simulink model "powertrain_control_3"  (R2026a)
settings: Solver=VariableStepAuto  StopTime=100  AbsTol=1e-3
PostLoadFcn:
  | num_fric_surf = 6;
  | eff_tor_rad = 0.4;
  | engagement_area = 0.0025;
  | peak_normal = 0.55;
  | fric_coeff = 0.5;
  | clutchRise = 0.1;
  | velTol = 1e-3;
  | pressThresh = 0.05;
  | p0 = 20e5;
undefined symbols (not defined in the file): sigbuilder_block
libraries: sdl_lib x13, fl_lib x11, nesl_utility x10
Description:
  | Copyright 2017-2026 The MathWorks, Inc.
settings Model: Creator=smiller  LastModifiedBy=smiller
settings ConfigComp: CovMetricSettings=dswe
settings SimscapeCC: SimscapeNormalizeSystem=off  SimscapeNominalValues="[{\"value\":\"1\",\"unit\":\"A\"},{\"value\":\"1\",\"unit\":\"bar\"},{\"value\":\"1\",\"unit\":\"cm^2\"},{\"value\":\"1\",\"unit\":\"cm^3/s\"},{\"value\":\"1\",\"unit\":\"kJ/kg\"},{\"value\":\"1\",\"unit\":\"kW\"},{\"value\":\"1\",\"unit\":\"l\"},{\"value\":\"1\",\"unit\":\"N\"},{\"value\":\"1\",\"unit\":\"N*m\"},{\"value\":\"1\",\"unit\":\"V\"}]"

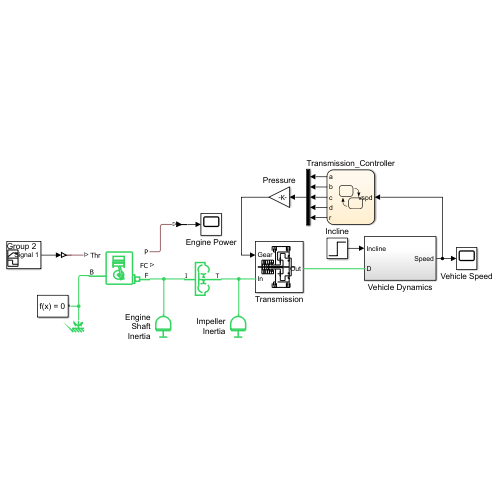
[thumbnail: Simulink's stored preview of the top-level diagram]
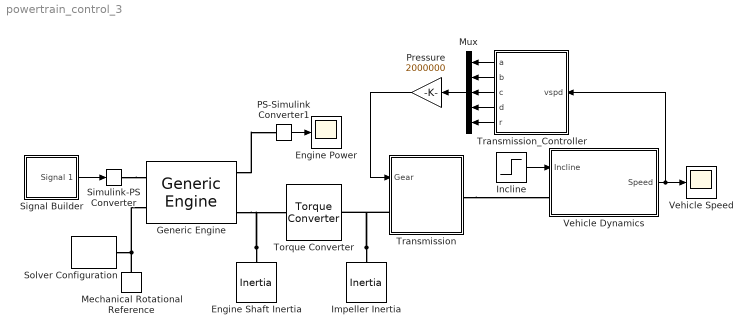
== system powertrain_control_3 ==
  Engine Shaft Inertia : fl_lib/Mechanical/Rotational Elements/Inertia  inertia=0.2 kg*m^2  num_ports=foundation.enum.numPorts2.one  w_specify=on  w_priority=High  w=800 rpm  w_nominal_specify=off  w_nominal_value=1  w_nominal_unit=rad/s  t_specify=off  t_priority=High  t=0 N*m  t_nominal_specify=off  t_nominal_value=1  t_nominal_unit=N*m
  Engine Power : Scope
      settings: ActiveDisplayYMinimum=-18750.18434  ActiveDisplayYMaximum=168751.65909
  Generic Engine : sdl_lib/Engines & Motors/Generic Engine  input_type=sdl.enum.GenericEngineInputType.NormalizedThrottle  model_parameterization=1  engine_type=1  Trq_max=380 N*m  w_Trq_max=4300 rpm  P_max=1.5e+5 W  w_P_max=4.5e+3 rpm  w_max=6e+3 rpm  w_min=500 rpm  w_tab=[ 500 1000 2e+3 3e+3 4e+3 5e+3 6e+3 7e+3 ] rpm  trq_tab=[ 380 380 380 380 350 280 200 80 ] N*m  pwr_tab=[ 2e+4 4e+4 7.8e+4 1.2e+5 1.45e+5 1.48e+5 1.25e+5 6e+4 ] W  interp_method=1  w_thr=100 rpm  model_inertia=0  inertia=1 kg*m^2  initial_velocity=800 rpm  model_time_constant=0  time_constant=0.2 s  initial_normalized_throttle=0  fc_model=1  fc_per_rev=25 mg/rev  fc_w_tab=[ 1000 2e+3 3e+3 4e+3 5e+3 6e+3 ] rpm  fc_trq_tab=[ 0 80 160 200 240 320 360 400 ] N*m  fc_tab=[ 0.5 0.9 1.4 1.6 1.9 2.7 3.4 4.4; 1 1.7 2.7 3.1 3.6 5 6 7.4; 1.4 2.7 4 4.8 5.6 7.5 8.5 10.5; 2 3.6 5.8 6.7 8 10.4 11.7 13.3; 2.5 4.8 7.9 9.4 10.8 14 16.2 18.6; 3.1 6 10.3 11.9 13.8 18.4 22 26.5 ] g/s  bmep_tab=[ 0 250 500 625 750 1000 1.15e+3 1.25e+3 ] kPa  bsfc_tab=[ 410 380 300 280 270 290 320 380; 410 370 290 270 260 270 285 320; 415 380 290 275 265 270 270 300; 420 390 310 290 285 280 280 285; 430 410 340 320 310 300 310 320; 450 430 370 340 330 330 350 380 ] g/hr/kW  fc_interp_method=1  displaced_volume=400 cm^3  rev_per_cycle=2  idle_speed=0  idle_speed_reference=1000 rpm  tau_controller=1 s  idle_w_thr=1 rpm  redline=0  redline_speed=5000 rpm  tau_redline=1 s  redline_w_thr=1 rpm
  Impeller Inertia : fl_lib/Mechanical/Rotational Elements/Inertia  inertia=1 kg*m^2  num_ports=foundation.enum.numPorts2.one  w_specify=on  w_priority=High  w=0 rpm  w_nominal_specify=off  w_nominal_value=1  w_nominal_unit=rad/s  t_specify=off  t_priority=High  t=0 N*m  t_nominal_specify=off  t_nominal_value=1  t_nominal_unit=N*m
  Incline : Step  Time=5  FinalValue=20  SampleTime=0
  Mechanical Rotational Reference : fl_lib/Mechanical/Rotational Elements/Mechanical Rotational Reference
  Mux : Mux  Inputs=5
  PS-Simulink Converter1 : nesl_utility/PS-Simulink Converter  PhysicalDomain=network_engine_domain  SubClassName=ps_output  LeftPortType=input  RightPortType=output  PseudoPeriodic=off  Frequencies=[]  VectorFormat=1-D array  Unit=W  AffineConversion=off
  Pressure : Gain  Gain=2000000
  Signal Builder : Subsystem  Tag=STV Subsys  LoadFcn=sigbuilder_block('load');  StartFcn=sigbuilder_block('start');  StopFcn=sigbuilder_block('stop');  ClipboardFcn=sigbuilder_block('clipboard');  mask(Sigbuilder block){tuvar=[0:10]}
      mask help: Simulink:masks:SigbuilderBlock_MD
      mask init:
      | if ~strcmp(get_param(bdroot(gcbh),'SimulationStatus'),'stopped') tuvar = sigbuilder_block('maskInit'); end
      settings: CopyFcn=sigbuilder_block('copy');  DeleteFcn=sigbuilder_block('delete');  ModelCloseFcn=sigbuilder_block('modelClose');  PreSaveFcn=sigbuilder_block('preSave');  PauseFcn=sigbuilder_block('pause');  ContinueFcn=sigbuilder_block('continue');  NameChangeFcn=sigbuilder_block('namechange');  OpenFcn=sigbuilder_block('open',[53.4 199.8 550.8 400.2 ]);  CloseFcn=sigbuilder_block('close');
      mask Display: plot(0, 0, 100, 100,[2, 2, 32, 32, 2], [68, 8, 8, 68, 68],[32, 2], [38, 38], [32, 19, 2],[53, 60, 44], [32, 17, 17, 2],[16, 16, 31, 31]);txt = getActiveGroup(gcbh);text(2, 100, txt,'verticalAlignment', 'top');
  Simulink-PS Converter : nesl_utility/Simulink-PS Converter  PhysicalDomain=network_engine_domain  SubClassName=ps_input  LeftPortType=input  RightPortType=output  PseudoPeriodic=off  Frequencies=[]  NoiseDistribution=none  NoiseParameters=[]  Unit=1  AffineConversion=off  FilteringAndDerivatives=zero  SimscapeFilterOrder=1  InputFilterTimeConstant=0.001  UdotUserProvided=1
  Solver Configuration : nesl_utility/Solver Configuration  PhysicalDomain=network_engine_domain  SubClassName=solver  LeftPortType=input  RightPortType=generic  Tones=[]  Harmonics=[]  SimulateNoise=off  Profile=off  UseLocalSampling=off  EnableSwitchedLinearOptims=on  FrequencyDomain=off  UseCCode=off  RelTol=0.001  AbsTol=1e-06  MinStep=1e-09  ToWorkspace=off  RevertToSquareIcSolve=off  NumHomotopyIterations=100  PhasorMode=off  PhasorModeNumHarmonics=1  ConsistencySolver=NEWTON_FTOL  CanonicalOrdering=UNORDERED  OptimizeIntermediates=UNOPTIMIZED  IndexReductionMethod=DerivativeReplacement  DoDC=off  ResidualTolerance=1e-9  ConsistencyTolSource=GLOBAL  ConsistencyAbsTol=0.001  ConsistencyRelTol=0.001  ConsistencyTolFactor=0.001  UseLocalSolver=off  LocalSolverChoice=NE_BACKWARD_EULER_ADVANCER  ResolveIndetEquations=on  FunctionEvalNumThread=1  LocalSolverSampleTime=.001  DoFixedCost=off  MaxNonlinIter=3  MaxModeIter=2  ComputeImpulses=off  ImpulseIterations=2  LinearAlgebra=Sparse  LinearAlgebraNumThread=0  EquationFormulation=NE_TIME_EF  DelaysMemoryBudget=1024  AutomaticFiltering=on  FilteringTimeConstant=0.001  PartitionStorageMethod=AS_NEEDED  PartitionMemoryBudget=1024  PartitionMethod=FAST  MultibodyUseLocalSolver=off  MultibodyLocalSolverChoice=ODE1  MultibodyLocalSolverSampleTime=0.001
  Torque Converter : sdl_lib/Couplings & Drives/Torque Converter  coast_mode_modeling=sdl.enum.torqueConverterContinuousTwomode.continuous  SR_drive_tlu=[0, .5, .6, .7, .8, .87, .92, .94, .96, .97, 1]  TR_drive_tlu=[2.232, 1.5462, 1.4058, 1.2746, 1.1528, 1.0732, 1.0192, 1, 1, 1, 1]  CF_drive_tlu=1e-4 * [.72558, .66322, .63463, .59042, .51331, .4144, .29287, .22444, .12186, .04386, 0] m*N/rpm^2  SR_coast_tlu=[0, .5, .6, .7, .8, .87, .92, .94, .96, .97, 1]  CF_coast_tlu=1e-4 * [.5079, .4643, .4442, .4133, .3593, .2901, .205, .1571, .0853, .0307, 0] m*N/rpm^2  iniMode=sdl.enum.torqueConverterInitialMode.drive  delta_w=1 rpm  n_vector=[ 0 0.5 0.6 0.7 0.8 0.81 0.82 0.83 0.84 0.85 0.86 0.87 0.88 0.89 0.9 0.92 0.94 0.96 0.97 ]  trq_vector=[ 2.232 1.5462 1.4058 1.2746 1.1528 1.1412 1.1296 1.1181 1.1067 1.0955 1.0843 1.0732 1.0622 1.0513 1.0405 1.0192 0.9983 0.9983 0.9983 ]  cf_vector_parameterization=1  cf_vector_reference_speed=1  cf_vector=[ 12.2938 12.8588 13.1452 13.6285 14.6163 14.7747 14.9516 15.1502 15.3748 15.6309 15.9253 16.2675 16.6698 17.1492 17.7298 19.3503 22.1046 29.9986 50 ] (rad/s)/(N*m)^0.5  cf_vector_sq=[ 0.006615999999999999 0.006048 0.005787 0.005384 0.004681 0.004581 0.004473 0.004357 0.00423 0.004093 0.003943 0.003779 0.003599 0.0034 0.003181 0.002671 0.002047 0.001111 4e-4 ] N*m/(rad/s)^2  interp_method=simscape.enum.interpolation.linear  extrap_method=simscape.enum.extrapolation.linear  model_lag=0  tau=0.02 s  initial_trq_ratio=0
  Transmission : Subsystem  Tag=PublishSubsystem  mask(CR-CR 4-Speed){}
      mask help: This is a template for a CR-CR 4-speed transmission. Copy it to your model, open it as a subsystem, and modify it for your use.
      settings: OpenFcn=open_system(gcbh,'force');
      mask Help: web(drive_help);
      mask Display:
      | % Icon data
      | Icon.x1 = [-1.3 -1.1 -1.1 -1 -1 -1 -0.9 -0.9 -0.9 -0.8 -0.8];
      | Icon.x1_1 = [-0.8 -0.7 -0.7 -0.7 -0.6 -0.6 -0.6 -0.5 -0.5 -0.5];
      | Icon.y1 = [0 0 0.15 0.15 0.05 0.15 0.15 0.05 0.15 0.15 0.05];
      | Icon.y1_1 =[0.15 0.15 0.05 0.15 0.15 0.07 0.15 0.15 0.07 0.15];
      | Icon.x2 = [-1.05 -1.05 -0.95 -0.95 -0.95 0.3];
      | Icon.y2 = [0.08   0     0     0.08  0    0];
      | Icon.x3 = [-0.85 -0.85 -0.75 -0.75 -0.75 0 0 -0.3 -0.3  0.3];
      | Icon.y3 = [0.08 0.02 0.02 0.08 0.02 0.02 0.15 0.15 0.33 0.33];
      | Icon.x3_1 = [-0.65 -0.65 -0.55 -0.55 -0.55 -0.4];
      | Icon.y3_1 = [0.1    0.05  0.05  0.1   0.05 0.05];
      | Icon.x4 = [-0.2 -0.1 -0.15 -0.15 -0.2 -0.1];
      | Icon.y4 = [0.12 0.12 0.12 0.18 0.18 0.18];
      | Icon.x5 = [-0.2 -0.1 -0.1 -0.15 -0.15 -0.4 -0.4];
      | Icon.y5 = [0.1 0.1 0.1 0.1 0.05 0.05 0.4];
      | Icon.x6 = [-0.2 -0.1 -0.15 -0.15 0.1 0.1 0.4 0.4];
      | Icon.y6 = [0.20 0.20 0.20 0.3 0.3 0.19 0.19 0];
      | Icon.x7 = [0.3 0.3 0.25 0.35];
      | Icon.y7 = [0 0.13 0.13 0.13];
      | Icon.x8 = [0.25 0.35 0.3 0.3 0.25 0.35];
      | Icon.y8 = [0.15 0.15 0.15 0.23 0.23 0.23];
      | Icon.x9 = [0.25 0.35 0.3 0.3];
      | Icon.y9 = [0.25 0.25 0.25 0.40];
      | Icon.x10 = [0.25 0.25 0.35 0.35 0.35 0.15 0.15 0.15];
      | Icon.y10 = [0.35 0.45 0.45 0.35 0.45 0.45 0.35 0.45];
      | Icon.x11 = [0.2 0.2];
      | Icon.y11 = [0.33 0.40];
      | Icon.x12 = [0.4 0.6];
      | Icon.y12 = [0 0];
      | Icon.x13 = [-0.45 -0.45 -0.35 -0.35 -0.35 -0.55 -0.55];
      | Icon.y13 = [0.35 0.45 0.45 0.35 0.45 0.45 0.35];
      | Icon.x14 = [-0.4 -0.5 -0.5];
      | Icon.y14 = [0.33 0.33 0.4];
      | Icon.x15 = [-0.5 0.35];
      | Icon.y15 = [0.45 0.45];
      | Icon.x16 = [-1.3 -1.1 -1.1 -1 -1 -1 -0.9 -0.9 ];
      | Icon.x16_1 = [-0.9 -0.8 -0.8 -0.8 -0.7 -0.7 -0.7 -0.6];
      | Icon.x16_2 = [-0.6 -0.6 -0.5 -0.5 -0.5];
      | Icon.y16 = [0 0 -0.15 -0.15 -0.05 -0.15 -0.15 -0.05];
      | Icon.y16_1 = [-0.15 -0.15 -0.05 -0.15 -0.15 -0.05 -0.15 -0.15];
      | Icon.y16_2 = [-0.07 -0.15 -0.15 -0.07 -0.15];
      | Icon.x17 = [-1.05 -1.05 -0.95 -0.95 -0.95 0.3];
      | Icon.y17 = [-0.08 0 0 -0.08 0 0];
      | Icon.x18 = [-0.85 -0.85 -0.75 -0.75 -0.75 0 0 -0.3];
      | Icon.x18_1 = [-0.3  0.3];
      | Icon.x18_2 = [-0.65 -0.65 -0.55 -0.55 -0.55 -0.4];
      | Icon.y18 = [-0.08 -0.02 -0.02 -0.08 -0.02 -0.02 -0.15 -0.15];
      | Icon.y18_1 = [-0.33 -0.33];
      | Icon.y18_2 = [-0.1 -0.05 -0.05 -0.1 -0.05 -0.05];
      | Icon.x19 = [-0.2 -0.1 -0.15 -0.15 -0.2 -0.1];
      | Icon.y19 = [-0.12 -0.12 -0.12 -0.18 -0.18 -0.18];
      | Icon.x20 = [-0.2 -0.1 -0.1 -0.15 -0.15 -0.4 -0.4];
      | Icon.y20 = [-0.1 -0.1 -0.1 -0.1 -0.05 -0.05 -0.4];
      | Icon.x21 = [-0.2 -0.1 -0.15 -0.15 0.1 0.1 0.4 0.4];
      | Icon.y21 = [-0.20 -0.20 -0.20 -0.3 -0.3 -0.19 -0.19 0];
      | Icon.x22 = [0.3 0.3 0.25 0.35];
      | Icon.y22 = [0 -0.13 -0.13 -0.13];
      | Icon.x23 = [0.25 0.35 0.3 0.3 0.25 0.35];
      | Icon.y23 = [-0.15 -0.15 -0.15 -0.23 -0.23 -0.23];
      | Icon.x24 = [0.25 0.35 0.3 0.3];
      | Icon.y24 = [-0.25 -0.25 -0.25 -0.40];
      | Icon.x25 = [0.25 0.25 0.35 0.35 0.35 0.15 0.15 0.15];
      | Icon.y25 = [-0.35 -0.45 -0.45 -0.35 -0.45 -0.45 -0.35 -0.45];
      | Icon.x26 = [0.2 0.2];
      | Icon.y26 = [-0.33 -0.40];
      | Icon.x27 = [-0.45 -0.45 -0.35 -0.35 -0.35 -0.55 -0.55];
      | Icon.y27 = [-0.35 -0.45 -0.45 -0.35 -0.45 -0.45 -0.35];
      | Icon.x28 = [-0.4 -0.5 -0.5];
      | Icon.y28 = [-0.33 -0.33 -0.4];
      | Icon.x29 = [-0.5 0.35];
      | Icon.y29 = [-0.45 -0.45];
      | % Bounding box
      | Icon.LowerLeftx = -1.4;
      | Icon.LowerLefty = -0.55;
      | Icon.UpperRightx = 1.0;
      | Icon.UpperRighty = 0.55;
      | 
      | plot(Icon.x1,Icon.y1);
      | plot(Icon.x1_1,Icon.y1_1);
      | plot(Icon.x2,Icon.y2);
      | plot(Icon.x3,Icon.y3);
      | plot(Icon.x3_1,Icon.y3_1);
      | plot(Icon.x4,Icon.y4);
      | plot(Icon.x5,Icon.y5);
      | plot(Icon.x6,Icon.y6);
      | plot(Icon.x7,Icon.y7);
      | plot(Icon.x8,Icon.y8);
      | plot(Icon.x9,Icon.y9);
      | plot(Icon.x10,Icon.y10);
      | plot(Icon.x11,Icon.y11);
      | plot(Icon.x12,Icon.y12);
      | plot(Icon.x13,Icon.y13);
      | plot(Icon.x14,Icon.y14);
      | plot(Icon.x15,Icon.y15);
      | plot(Icon.x16,Icon.y16);
      | plot(Icon.x16_1,Icon.y16_1);
      | plot(Icon.x16_2,Icon.y16_2);
      | plot(Icon.x17,Icon.y17);
      | plot(Icon.x18,Icon.y18);
      | plot(Icon.x18_1,Icon.y18_1);
      | plot(Icon.x18_2,Icon.y18_2);
      | plot(Icon.x19,Icon.y19);
      | plot(Icon.x20,Icon.y20);
      | plot(Icon.x21,Icon.y21);
      | plot(Icon.x22,Icon.y22);
      | plot(Icon.x23,Icon.y23);
      | plot(Icon.x24,Icon.y24);
      | plot(Icon.x25,Icon.y25);
      | plot(Icon.x26,Icon.y26);
      | plot(Icon.x27,Icon.y27);
      | plot(Icon.x28,Icon.y28);
      | plot(Icon.x29,Icon.y29);
      | 
      | plot(Icon.LowerLeftx,Icon.LowerLefty);
      | plot(Icon.UpperRightx,Icon.UpperRighty);
  Transmission_Controller : Stateflow chart  TreatAsAtomicUnit=on
  Vehicle Dynamics : Subsystem
  Vehicle Speed : Scope
      settings: ActiveDisplayYMinimum=-12.57055  ActiveDisplayYMaximum=113.13493
  wires:
  Vehicle Dynamics/1(Speed) -> Transmission_Controller/1(vspd), Vehicle Speed/1
  PS-Simulink Converter1/1 -> Engine Power/1
  Incline/1 -> Vehicle Dynamics/1(Incline)
  Transmission_Controller/1(a) -> Mux/1
  Transmission_Controller/2(b) -> Mux/2
  Transmission_Controller/3(c) -> Mux/3
  Transmission_Controller/4(d) -> Mux/4
  Transmission_Controller/5(r) -> Mux/5
  Mux/1 -> Pressure/1
  Pressure/1 -> Transmission/1(Gear)
  Signal Builder/1(Signal 1) -> Simulink-PS Converter/1
  connections:
  Solver Configuration/RConn1 -- Mechanical Rotational Reference/LConn1 -- Generic Engine/LConn2
  Impeller Inertia/LConn1 -- Transmission/LConn1 -- Torque Converter/RConn1
  Engine Shaft Inertia/LConn1 -- Torque Converter/LConn1 -- Generic Engine/RConn3
  Transmission/RConn1 -- Vehicle Dynamics/LConn1
  Generic Engine/RConn1 -- PS-Simulink Converter1/LConn1
  Simulink-PS Converter/RConn1 -- Generic Engine/LConn1

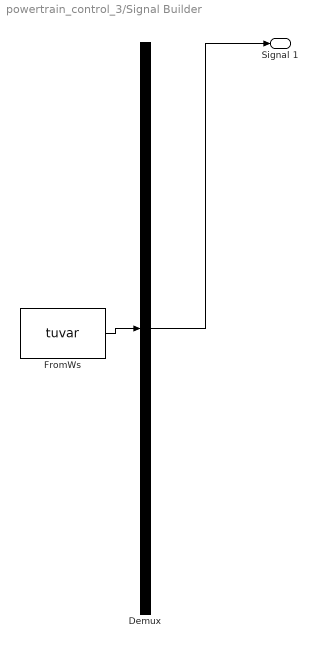
== system powertrain_control_3/Signal Builder ==
  Demux : Demux  Tag=STV Demux  Outputs=1
      settings: DisplayOption=none
  FromWs : FromWorkspace  Tag=STV FromWs  VariableName=tuvar
      SigBuilderData=|
      | common.afterFinalStr = 'Extrapolate'
      | common.sampleTime = 0
      | dataSet(1).timeRange = [0 100]
      | dataSet(1).name = 'Group 1'
      | dataSet(2).timeRange = [0 100]
      | dataSet(2).name = 'Group 2'
      | sbobj.Groups(1).Name = 'Group 1'
      | sbobj.Groups(1).Signals.Name = 'Signal 1'
      | sbobj.Groups(1).Signals.XData = [0 100]
      | sbobj.Groups(1).Signals.YData = [1 1]
      | sbobj.Groups(1).TimeRange = [0 100]
      | sbobj.Groups(2).Name = 'Group 2'
      | sbobj.Groups(2).Signals.Name = 'Signal 1'
      | sbobj.Groups(2).Signals.XData = [0 40 40 100]
      | sbobj.Groups(2).Signals.YData = [0.5 0.5 1 1]
      | sbobj.Groups(2).TimeRange = [0 100]
  Signal 1 : Outport  Tag=STV Outport  VectorParamsAs1DForOutWhenUnconnected=off
  wires:
  Demux/1 -> Signal 1/1
  FromWs/1 -> Demux/1

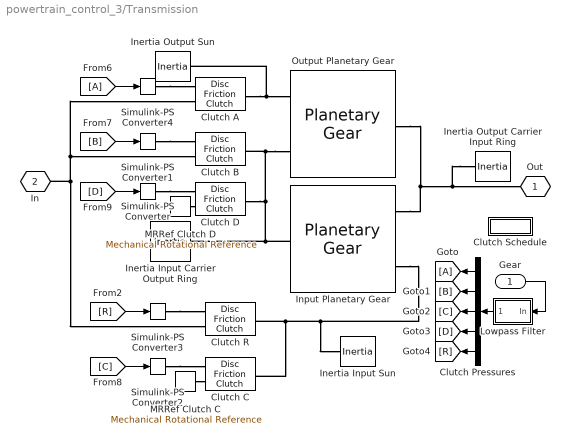
== system powertrain_control_3/Transmission ==
  Gear : Inport
  Clutch Pressures : Demux  Outputs=5
  Clutch A : sdl_lib/Clutches/Disc Friction Clutch  geometry_model=1  r_eff=eff_tor_rad m  d_o=0.15 m  d_i=0.1 m  nS=num_fric_surf  piston_area=engagement_area m^2  unidirectional=0  friction_model=1  mu_w_vector=[ 0 0.1 0.2 0.3 0.4 0.5 1 2 5 10 100 1000 ] rad/s  temperature_TLU=[280.0, 300.0, 320.0] K  mu_static=peak_normal  mu_static_vector=[0.4, 0.38, 0.36]  mu_coulomb=fric_coeff  mu_coulomb_vector=[ 0.29 0.28 0.26 0.22 0.21 0.2 0.2 0.19 0.19 0.19 0.19 0.19 ]  mu_coulomb_temp_vector=[0.3, 0.28, 0.25]  mu_coulomb_matrix=[0.34, 0.32, 0.3; 0.3, 0.28, 0.25; 0.25, 0.2, 0.15]  mu_interp_method=1  mu_extrap_method=1  d_f=1  w_tol=velTol rad/s  pressure_min=pressThresh*p0 Pa  mu_visc=0 N*m/(rad/s)  initial_state_locked=1  thermal_mass=25 kJ/K  T_init=300 K
  Clutch B : sdl_lib/Clutches/Disc Friction Clutch  geometry_model=1  r_eff=eff_tor_rad m  d_o=0.15 m  d_i=0.1 m  nS=num_fric_surf  piston_area=engagement_area m^2  unidirectional=0  friction_model=1  mu_w_vector=[ 0 0.1 0.2 0.3 0.4 0.5 1 2 5 10 100 1000 ] rad/s  temperature_TLU=[280.0, 300.0, 320.0] K  mu_static=peak_normal  mu_static_vector=[0.4, 0.38, 0.36]  mu_coulomb=fric_coeff  mu_coulomb_vector=[ 0.29 0.28 0.26 0.22 0.21 0.2 0.2 0.19 0.19 0.19 0.19 0.19 ]  mu_coulomb_temp_vector=[0.3, 0.28, 0.25]  mu_coulomb_matrix=[0.34, 0.32, 0.3; 0.3, 0.28, 0.25; 0.25, 0.2, 0.15]  mu_interp_method=1  mu_extrap_method=1  d_f=1  w_tol=velTol rad/s  pressure_min=pressThresh*p0 Pa  mu_visc=0 N*m/(rad/s)  initial_state_locked=0  thermal_mass=25 kJ/K  T_init=300 K
  Clutch C : sdl_lib/Clutches/Disc Friction Clutch  geometry_model=1  r_eff=eff_tor_rad m  d_o=0.15 m  d_i=0.1 m  nS=num_fric_surf  piston_area=engagement_area m^2  unidirectional=0  friction_model=1  mu_w_vector=[ 0 0.1 0.2 0.3 0.4 0.5 1 2 5 10 100 1000 ] rad/s  temperature_TLU=[280.0, 300.0, 320.0] K  mu_static=peak_normal  mu_static_vector=[0.4, 0.38, 0.36]  mu_coulomb=fric_coeff  mu_coulomb_vector=[ 0.29 0.28 0.26 0.22 0.21 0.2 0.2 0.19 0.19 0.19 0.19 0.19 ]  mu_coulomb_temp_vector=[0.3, 0.28, 0.25]  mu_coulomb_matrix=[0.34, 0.32, 0.3; 0.3, 0.28, 0.25; 0.25, 0.2, 0.15]  mu_interp_method=1  mu_extrap_method=1  d_f=1  w_tol=velTol rad/s  pressure_min=pressThresh*p0 Pa  mu_visc=0 N*m/(rad/s)  initial_state_locked=0  thermal_mass=25 kJ/K  T_init=300 K
  Clutch D : sdl_lib/Clutches/Disc Friction Clutch  geometry_model=1  r_eff=eff_tor_rad m  d_o=0.15 m  d_i=0.1 m  nS=num_fric_surf  piston_area=engagement_area m^2  unidirectional=0  friction_model=1  mu_w_vector=[ 0 0.1 0.2 0.3 0.4 0.5 1 2 5 10 100 1000 ] rad/s  temperature_TLU=[280.0, 300.0, 320.0] K  mu_static=peak_normal  mu_static_vector=[0.4, 0.38, 0.36]  mu_coulomb=fric_coeff  mu_coulomb_vector=[ 0.29 0.28 0.26 0.22 0.21 0.2 0.2 0.19 0.19 0.19 0.19 0.19 ]  mu_coulomb_temp_vector=[0.3, 0.28, 0.25]  mu_coulomb_matrix=[0.34, 0.32, 0.3; 0.3, 0.28, 0.25; 0.25, 0.2, 0.15]  mu_interp_method=1  mu_extrap_method=1  d_f=1  w_tol=velTol rad/s  pressure_min=pressThresh*p0 Pa  mu_visc=0 N*m/(rad/s)  initial_state_locked=1  thermal_mass=25 kJ/K  T_init=300 K
  Clutch R : sdl_lib/Clutches/Disc Friction Clutch  geometry_model=1  r_eff=eff_tor_rad m  d_o=0.15 m  d_i=0.1 m  nS=num_fric_surf  piston_area=engagement_area m^2  unidirectional=0  friction_model=1  mu_w_vector=[ 0 0.1 0.2 0.3 0.4 0.5 1 2 5 10 100 1000 ] rad/s  temperature_TLU=[280.0, 300.0, 320.0] K  mu_static=peak_normal  mu_static_vector=[0.4, 0.38, 0.36]  mu_coulomb=fric_coeff  mu_coulomb_vector=[ 0.29 0.28 0.26 0.22 0.21 0.2 0.2 0.19 0.19 0.19 0.19 0.19 ]  mu_coulomb_temp_vector=[0.3, 0.28, 0.25]  mu_coulomb_matrix=[0.34, 0.32, 0.3; 0.3, 0.28, 0.25; 0.25, 0.2, 0.15]  mu_interp_method=1  mu_extrap_method=1  d_f=1  w_tol=velTol rad/s  pressure_min=pressThresh*p0 Pa  mu_visc=0 N*m/(rad/s)  initial_state_locked=0  thermal_mass=25 kJ/K  T_init=300 K
  Clutch Schedule : Subsystem  Tag=PublishSubsystem
  From6 : From
      settings: CloseFcn=tagdialog Close
  Goto : Goto
  Inertia Input Sun : fl_lib/Mechanical/Rotational Elements/Inertia  inertia=1e-4 kg*m^2  num_ports=foundation.enum.numPorts2.one  w_specify=on  w_priority=High  w=0 rad/s  w_nominal_specify=off  w_nominal_value=1  w_nominal_unit=rad/s  t_specify=off  t_priority=High  t=0 N*m  t_nominal_specify=off  t_nominal_value=1  t_nominal_unit=N*m
  Inertia Input Carrier Output Ring : fl_lib/Mechanical/Rotational Elements/Inertia  inertia=1e-4 kg*m^2  num_ports=foundation.enum.numPorts2.one  w_specify=on  w_priority=High  w=0 rad/s  w_nominal_specify=off  w_nominal_value=1  w_nominal_unit=rad/s  t_specify=off  t_priority=High  t=0 N*m  t_nominal_specify=off  t_nominal_value=1  t_nominal_unit=N*m
  Inertia Output Carrier Input Ring : fl_lib/Mechanical/Rotational Elements/Inertia  inertia=1e-4 kg*m^2  num_ports=foundation.enum.numPorts2.one  w_specify=on  w_priority=High  w=0 rad/s  w_nominal_specify=off  w_nominal_value=1  w_nominal_unit=rad/s  t_specify=off  t_priority=High  t=0 N*m  t_nominal_specify=off  t_nominal_value=1  t_nominal_unit=N*m
  Inertia Output Sun : fl_lib/Mechanical/Rotational Elements/Inertia  inertia=1e-4 kg*m^2  num_ports=foundation.enum.numPorts2.one  w_specify=on  w_priority=High  w=0 rad/s  w_nominal_specify=off  w_nominal_value=1  w_nominal_unit=rad/s  t_specify=off  t_priority=High  t=0 N*m  t_nominal_specify=off  t_nominal_value=1  t_nominal_unit=N*m
  "Input Planetary Gear " : sdl_lib/Gears/Planetary Gear  rs_ratio=2.2258  friction_model=1  efficiency=[ 0.96 0.98 ]  temperature_TLU=[ 280 300 320 ] K  efficiency_sp_TLU=[ 0.95 0.9 0.85 ]  efficiency_rp_TLU=[ 0.95 0.9 0.85 ]  pwr_thr=[ 0.001 0.001 ] W  mu_visc=[ 0 0 ] N*m/(rad/s)  model_inertia=0  sun_inertia=1e-10 kg*m^2  ring_inertia=1e-10 kg*m^2  carrier_inertia=1e-10 kg*m^2  carrier_radius=0.01 m  planet_inertia=0.001 kg*m^2  planet_mass=1e-10 kg  thermal_mass=50 J/K  T_init=300 K
  Lowpass Filter : Subsystem  mask(First-order lag supporting vector signals){b=0.05, x_initial=[0 0 0 0 0]}
      mask prompts: b "Filter time constant"; x_initial "Initial output"
      mask help: Models a lag of the form 1/(b*s+1) where s is the Laplace operator.
  MRRef Clutch C : fl_lib/Mechanical/Rotational Elements/Mechanical Rotational Reference
  MRRef Clutch D : fl_lib/Mechanical/Rotational Elements/Mechanical Rotational Reference
  Output Planetary Gear : sdl_lib/Gears/Planetary Gear  rs_ratio=1.84  friction_model=1  efficiency=[ 0.96 0.98 ]  temperature_TLU=[ 280 300 320 ] K  efficiency_sp_TLU=[ 0.95 0.9 0.85 ]  efficiency_rp_TLU=[ 0.95 0.9 0.85 ]  pwr_thr=[ 0.001 0.001 ] W  mu_visc=[0 0] N*m/(rad/s)  model_inertia=0  sun_inertia=1e-10 kg*m^2  ring_inertia=1e-10 kg*m^2  carrier_inertia=1e-10 kg*m^2  carrier_radius=0.01 m  planet_inertia=0.001 kg*m^2  planet_mass=1e-10 kg  thermal_mass=50 J/K  T_init=300 K
  Simulink-PS Converter{,1..4} (5 alike) : nesl_utility/Simulink-PS Converter  PhysicalDomain=network_engine_domain  SubClassName=ps_input  LeftPortType=input  RightPortType=output  PseudoPeriodic=off  Frequencies=[]  NoiseDistribution=none  NoiseParameters=[]  Unit=1  AffineConversion=off  FilteringAndDerivatives=zero  SimscapeFilterOrder=1  InputFilterTimeConstant=.001  UdotUserProvided=0
  Out : PMIOPort  Tag=PMCPort  Side=Right
  In : PMIOPort  Tag=PMCPort  Port=2  Side=Left
  wires:
  Gear/1 -> Lowpass Filter/1(In)
  Lowpass Filter/1(Out) -> Clutch Pressures/1
  Clutch Pressures/1 -> Goto/1
  Clutch Pressures/2 -> [B]
  Clutch Pressures/3 -> [C]
  Clutch Pressures/4 -> [D]
  Clutch Pressures/5 -> [R]
  [D] -> Simulink-PS Converter/1
  [B] -> Simulink-PS Converter1/1
  [C] -> Simulink-PS Converter2/1
  [R] -> Simulink-PS Converter3/1
  From6/1 -> Simulink-PS Converter4/1
  connections:
  Inertia Output Carrier Input Ring/LConn1 -- Out/RConn1 -- "Input Planetary Gear "/RConn1 -- Output Planetary Gear/LConn1
  Inertia Output Sun/LConn1 -- Output Planetary Gear/RConn2 -- Clutch A/RConn1
  MRRef Clutch D/LConn1 -- Clutch D/LConn2
  Simulink-PS Converter/RConn1 -- Clutch D/LConn1
  Clutch R/RConn1 -- Inertia Input Sun/LConn1 -- "Input Planetary Gear "/RConn2 -- Clutch C/RConn1
  Output Planetary Gear/RConn1 -- Clutch B/RConn1 -- Clutch D/RConn1 -- Inertia Input Carrier Output Ring/LConn1 -- "Input Planetary Gear "/LConn1
  Simulink-PS Converter1/RConn1 -- Clutch B/LConn1
  In/RConn1 -- Clutch B/LConn2 -- Clutch A/LConn2 -- Clutch R/LConn2
  MRRef Clutch C/LConn1 -- Clutch C/LConn2
  Simulink-PS Converter2/RConn1 -- Clutch C/LConn1
  Simulink-PS Converter3/RConn1 -- Clutch R/LConn1
  Simulink-PS Converter4/RConn1 -- Clutch A/LConn1

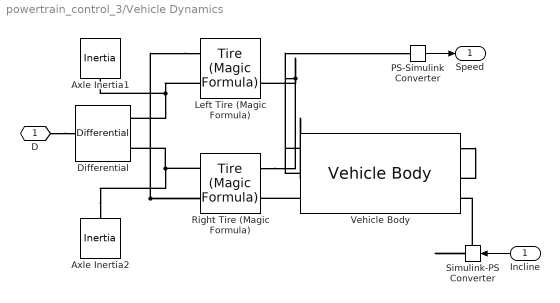
== system powertrain_control_3/Vehicle Dynamics ==
  Incline : Inport
  Axle Inertia1 : fl_lib/Mechanical/Rotational Elements/Inertia  inertia=1 kg*m^2  num_ports=foundation.enum.numPorts2.one  w_specify=on  w_priority=High  w=0 rad/s  w_nominal_specify=off  w_nominal_value=1  w_nominal_unit=rad/s  t_specify=off  t_priority=High  t=0 N*m  t_nominal_specify=off  t_nominal_value=1  t_nominal_unit=N*m
  Axle Inertia2 : fl_lib/Mechanical/Rotational Elements/Inertia  inertia=1 kg*m^2  num_ports=foundation.enum.numPorts2.one  w_specify=on  w_priority=High  w=0 rad/s  w_nominal_specify=off  w_nominal_value=1  w_nominal_unit=rad/s  t_specify=off  t_priority=High  t=0 N*m  t_nominal_specify=off  t_nominal_value=1  t_nominal_unit=N*m
  Differential : sdl_lib/Gears/Differential  driveshaft_location=2  cd_ratio=4  friction_model=1  efficiency=[ 0.85 0.92 ]  temperature_TLU=[ 280 300 320 ] K  efficiency_ss_TLU=[ 0.95 0.9 0.85 ]  efficiency_cd_TLU=[ 0.95 0.9 0.85 ]  pwr_thr=[ 0.001 0.001 ] W  mu_visc=[ 0 0 ] N*m/(rad/s)  model_inertia=0  sun_inertia=1e-10 kg*m^2  sun_radius=0.01 m  carrier_inertia=0.001 kg*m^2  planet_inertia=0.001 kg*m^2  planet_mass=1e-10 kg  thermal_mass=50 J/K  T_init=300 K
  Left Tire (Magic Formula) : sdl_lib/Tires & Vehicles/Tire (Magic Formula)  parameterization=1  F_z1=3e+3 N  F_x1=3.5e+3 N  kappa1=10  B_m=10  C_m=1.9  D_m=1  E_m=0.97  fz0=4e+3 N  p_Cx=1.685  p_Dx=[ 1.21 -0.037 ]  p_Ex=[ 0.344 0.095 -0.02 0 ]  p_Kx=[ 21.51 -0.163 0.245 ]  p_Hx=[ -0.002 0.002 ]  p_Vx=[ 0 0 ]  rolling_radius_model=sdl.enum.RollingRadiusParameterization.Constant  r_e=0.3 m  r_0=0.3 m  breff=8.39  dreff=0.26  freff=0.074  q_re0=0.99  q_v1=0.008  longvl=17 m/s  cz=5e5 N/m  model_resistance=0  resistance_model=1  coeff=0.015  p_tire=250e3 Pa  alpha=-0.003  beta=0.97  coeff_a=84e-4  coeff_b=6.2e-4 s/m  coeff_c=1.6e-4 s^2/m^2  p_tire0=240e3 Pa  fz0_resistance=4000 N  vH0=16 m/s  q_Sy=[.0082, 0, .0014, .001, 0, 0, 1.08, -.5]  v_thr=1e-3 m/s  enable_scaling_coefficients=false  lfzO=1  lcx=1  lmux=1  lex=1  lkx=1  lhx=1  lvx=1  lmy=1  model_compliance=0  stiffness=1e+6 N/m  damping=1000 N/(m/s)  model_inertia=0  inertia=1 kg*m^2  initial_velocity=0 rad/s  vxlow=0.1 m/s  v_tr_thr=0.1*(0.1) m/s  kpumin=-1e5  kpumax=1e5
  PS-Simulink Converter : nesl_utility/PS-Simulink Converter  PhysicalDomain=network_engine_domain  SubClassName=ps_output  LeftPortType=input  RightPortType=output  PseudoPeriodic=off  Frequencies=[]  VectorFormat=1-D array  Unit=km/hr  AffineConversion=off
  Right Tire (Magic Formula) : sdl_lib/Tires & Vehicles/Tire (Magic Formula)  parameterization=1  F_z1=3e+3 N  F_x1=3.5e+3 N  kappa1=10  B_m=10  C_m=1.9  D_m=1  E_m=0.97  fz0=4e+3 N  p_Cx=1.685  p_Dx=[ 1.21 -0.037 ]  p_Ex=[ 0.344 0.095 -0.02 0 ]  p_Kx=[ 21.51 -0.163 0.245 ]  p_Hx=[ -0.002 0.002 ]  p_Vx=[ 0 0 ]  rolling_radius_model=sdl.enum.RollingRadiusParameterization.Constant  r_e=0.3 m  r_0=0.3 m  breff=8.39  dreff=0.26  freff=0.074  q_re0=0.99  q_v1=0.008  longvl=17 m/s  cz=5e5 N/m  model_resistance=0  resistance_model=1  coeff=0.015  p_tire=250e3 Pa  alpha=-0.003  beta=0.97  coeff_a=84e-4  coeff_b=6.2e-4 s/m  coeff_c=1.6e-4 s^2/m^2  p_tire0=240e3 Pa  fz0_resistance=4000 N  vH0=16 m/s  q_Sy=[.0082, 0, .0014, .001, 0, 0, 1.08, -.5]  v_thr=1e-3 m/s  enable_scaling_coefficients=false  lfzO=1  lcx=1  lmux=1  lex=1  lkx=1  lhx=1  lvx=1  lmy=1  model_compliance=0  stiffness=1e+6 N/m  damping=1000 N/(m/s)  model_inertia=0  inertia=1 kg*m^2  initial_velocity=0 rad/s  vxlow=0.1 m/s  v_tr_thr=0.1*(0.1) m/s  kpumin=-1e5  kpumax=1e5
  Simulink-PS Converter : nesl_utility/Simulink-PS Converter  PhysicalDomain=network_engine_domain  SubClassName=ps_input  LeftPortType=input  RightPortType=output  PseudoPeriodic=off  Frequencies=[]  NoiseDistribution=none  NoiseParameters=[]  Unit=deg  AffineConversion=off  FilteringAndDerivatives=zero  SimscapeFilterOrder=1  InputFilterTimeConstant=.001  UdotUserProvided=0
  Vehicle Body : sdl_lib/Tires & Vehicles/Vehicle Body  mass=1.2e+3 kg  n_w=2  x_f=1.4 m  x_r=1.6 m  y_c=0.5 m  mass_var=simscape.enum.onoff.off  g=9.81 m/s^2  liftoff_warning=0  area=3 m^2  Cd_var=false  Cd=0.4  rho=1.18 kg/m^3  model_pitch=0  inertia=4000 kg*m^2  suspension_model=1  k_f=1e4 N/m  b_f=1e4 N/(m/s)  k_r=1e4 N/m  b_r=1e4 N/(m/s)  k_f_TLU=[-2000, -1000, 0, 1000, 2000] N  x_f_TLU=[-.4, -.2, 0, .2, .4] m  b_f_TLU=[-200, -100, 0, 100, 200] N  v_f_TLU=[-4, -2, 0, 2, 4] m/s  k_r_TLU=[-2000, -1000, 0, 1000, 2000] N  x_r_TLU=[-.4, -.2, 0, .2, .4] m  b_r_TLU=[-200, -100, 0, 100, 200] N  v_r_TLU=[-4, -2, 0, 2, 4] m/s  interp_method=simscape.enum.interpolation.linear  extrap_method=simscape.enum.extrapolation.linear  model_hardstop=0  upper_bound_f=.25 m  lower_bound_f=-.25 m  stop_k_f=1e6 N/m  stop_b_f=150 N/(m/s)  upper_bound_r=.25 m  lower_bound_r=-.25 m  stop_k_r=1e6 N/m  stop_b_r=150 N/(m/s)  initial_pitch=0 rad  initial_pitch_rate=0 rad/s  v_specify=on  v_priority=High  v=0 m/s  v_nominal_specify=off  v_nominal_value=1  v_nominal_unit=m/s
  D : PMIOPort  Side=Left
  Speed : Outport  VectorParamsAs1DForOutWhenUnconnected=off
  wires:
  PS-Simulink Converter/1 -> Speed/1
  Incline/1 -> Simulink-PS Converter/1
  connections:
  Axle Inertia1/LConn1 -- Left Tire (Magic Formula)/LConn2 -- Differential/RConn2
  Axle Inertia2/LConn1 -- Right Tire (Magic Formula)/LConn2 -- Differential/RConn1
  Left Tire (Magic Formula)/LConn1 -- Vehicle Body/RConn1 -- Right Tire (Magic Formula)/LConn1
  Vehicle Body/LConn1 -- Right Tire (Magic Formula)/RConn2 -- Left Tire (Magic Formula)/RConn2
  Vehicle Body/LConn2 -- PS-Simulink Converter/LConn1
  Simulink-PS Converter/RConn1 -- Vehicle Body/RConn3
  D/RConn1 -- Differential/LConn1

== system powertrain_control_3/Transmission/Clutch Schedule ==
  note: Clutch Schedule
  note: 0 - Disengaged, 1 - Engaged
  note: g1: Input planetary ring/sun gear ratio
      | g2: Output planetary ring/sun gear ratio
  note: Gear
      | A
      | B
      | C
      | D
      | R
      | Ratio
      |
      | R
      | 0
      | 0
      | 0
      | 1
      | 1
      | -g1
      |
      | 1
      | 1
      | 0
      | 0
      | 1
      | 0
      | g2
      |
      | 2
      | 1
      | 0
      | 1
      | 0
      | 0
      | (g1+g2)/(1+g1)
      |
      | 3
      | 1
      | 1
      | 0
      | 0
      | 0
      | 1
      |
      | 4
      | 0
      | 1
      | 1
      | 0
      | 0
      | g1 /(1+g1)

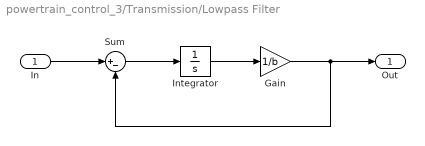
== system powertrain_control_3/Transmission/Lowpass Filter ==
  In : Inport
  Gain : Gain  Gain=1/b
  Integrator : Integrator  InitialCondition=x_initial*b
  Sum : Sum  Inputs=|+-  InputSameDT=on  SaturateOnIntegerOverflow=on  OutDataTypeStr=Inherit: Same as first input
  Out : Outport  VectorParamsAs1DForOutWhenUnconnected=off
  wires:
  Gain/1 -> Out/1, Sum/2
  Integrator/1 -> Gain/1
  In/1 -> Sum/1
  Sum/1 -> Integrator/1

== stateflow chart powertrain_control_3/Transmission_Controller ==
  state first
    entry: a=1;
    b=0;
    c=0;
    d=1;
    r=0;
  state third
    entry: a=1;
    b=1;
    c=0;
    d=0;
    r=0;
  state second
    entry: a=1;
    b=0;
    c=1;
    d=0;
    r=0;
  state fourth
    entry: a=0;
    b=1;
    c=1;
    d=0;
    r=0;
  third -> fourth [order 1] : [vspd>100]
  first -> second : [vspd>30]
  second -> third [order 1] : [vspd>65]
  (default) -> first
  second -> first [order 2] : [vspd<20]
  third -> second [order 2] : [vspd<55]
  fourth -> third : [vspd<90]
  data: vspd input; a output double; b output double; c output double; d output double; r output double
